simulink model "robotracer_simulation_gazebo"  (R2020a)
settings: Solver=VariableStepAuto  StartTime=0.0  StopTime=10  RelTol=1e-3
libraries: robotgazebolib x2, simulink x1
settings Model: Creator=under  LastModifiedBy=under

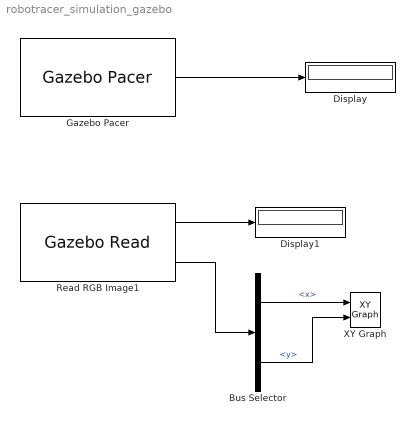
== system robotracer_simulation_gazebo ==
  Bus Selector : BusSelector  OutputSignals=position.x,position.y
  Display : Display
  Display1 : Display
  Gazebo Pacer : robotgazebolib/Gazebo Pacer  ResetBehavior=Reset Gazebo simulation time and scene  SampleTime=0.01
      settings: SourceProductBaseCode=RO
  Read RGB Image1 : robotgazebolib/Gazebo Read  topicSource=From Gazebo  topic=/gazebo/ground_truth/world_pose/robotracer_v1/base_link  messageType=gazebo_msgs/Pose  sampleTime=0.1
      settings: SourceProductBaseCode=RO
  XY Graph : simulink/Sinks/XY Graph  xmin=-5  xmax=5  ymin=-5  ymax=5  st=-1
  wires:
  Gazebo Pacer/1 -> Display/1
  Read RGB Image1/1 -> Display1/1
  Read RGB Image1/2 -> Bus Selector/1
  Bus Selector/1 -> XY Graph/1  "<x>"
  Bus Selector/2 -> XY Graph/2  "<y>"
